simulink model "Observer"  (R2022a)
settings: Solver=VariableStepAuto  StartTime=0.0  StopTime=30.0  RelTol=1e-3
settings Model: Creator=anthony  LastModifiedBy=anthony

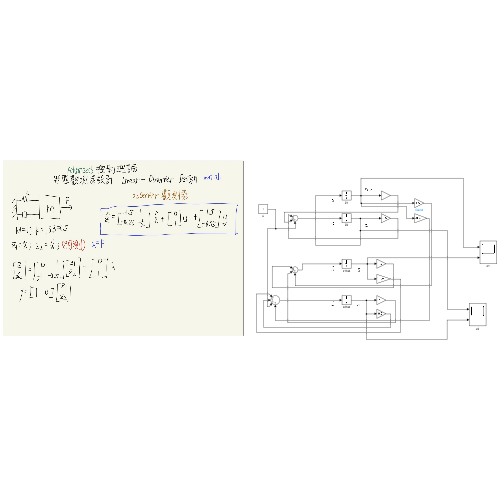
[thumbnail: Simulink's stored preview of the top-level diagram]
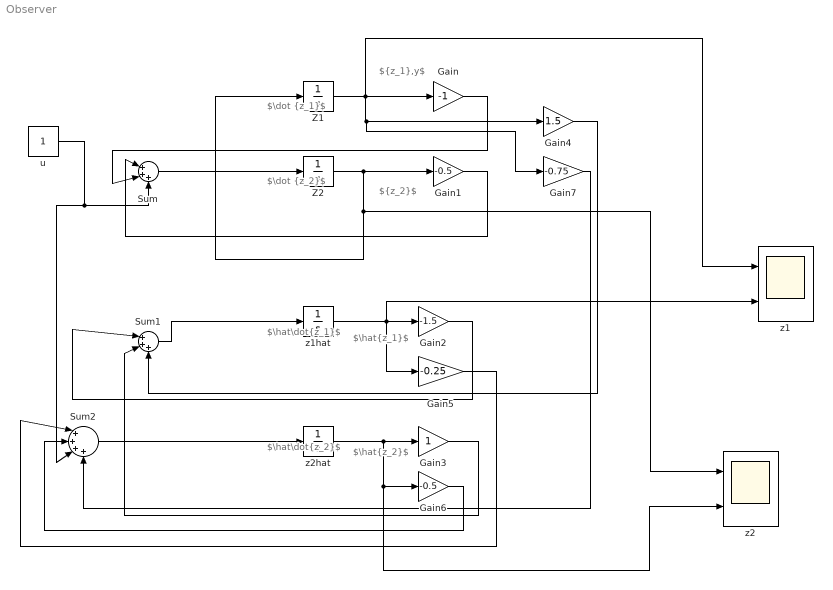
== system Observer ==
  note: $\dot {z_1}$
  note: $\dot {z_2}$
  note: ${z_1},y$
  note: $\hat{z_1}$
  note: $\hat\dot{z_1}$
  note: $\hat{z_2}$
  note: $\hat\dot{z_2}$
  note: ${z_2}$
  Gain : Gain  Gain=-1
  Gain1 : Gain  Gain=-0.5
  Gain2 : Gain  Gain=-1.5
  Gain3 : Gain
  Gain4 : Gain  Gain=1.5
  Gain5 : Gain  Gain=-0.25
  Gain6 : Gain  Gain=-0.5
  Gain7 : Gain  Gain=-0.75
  Sum : Sum  Inputs=|+++
  Sum1 : Sum  Inputs=|+++
  Sum2 : Sum  Inputs=|++++
  Z1 : Integrator
  Z2 : Integrator
  u : Constant
  z1 : Scope  NumInputPorts=2
  z1hat : Integrator
  z2 : Scope  NumInputPorts=2
  z2hat : Integrator  InitialCondition=1
  wires:
  Sum/1 -> Z2/1
  Z1/1 -> Gain/1, z1/1, Gain7/1, Gain4/1
  Gain/1 -> Sum/2
  Z2/1 -> Gain1/1, z2/1, Z1/1
  Gain1/1 -> Sum/1
  u/1 -> Sum2/3, Sum/3
  Sum1/1 -> z1hat/1
  z1hat/1 -> z1/2, Gain5/1, Gain2/1
  Gain2/1 -> Sum1/1
  z2hat/1 -> z2/2, Gain6/1, Gain3/1
  Gain3/1 -> Sum1/2
  Gain4/1 -> Sum1/3
  Sum2/1 -> z2hat/1
  Gain5/1 -> Sum2/1
  Gain6/1 -> Sum2/2
  Gain7/1 -> Sum2/4
